simulink model "position_interface"  (R2019b)
settings: Solver=VariableStepAuto  StartTime=0.0  StopTime=10.0  RelTol=1e-3
undefined symbols (not defined in the file or in its folder): Kd, Ki, Kp
settings Model: Creator=AL30832  LastModifiedBy=AL30832

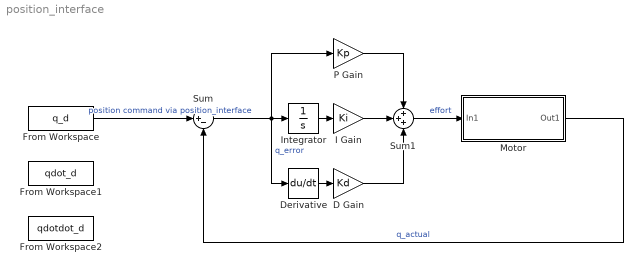
== system position_interface ==
  D Gain : Gain  Gain=Kd
  Derivative : Derivative  CoefficientInTFapproximation=Derivative
  From Workspace : FromWorkspace  VariableName=q_d  SampleTime=0
  From Workspace1 : FromWorkspace  VariableName=qdot_d  SampleTime=0
  From Workspace2 : FromWorkspace  VariableName=qdotdot_d  SampleTime=0
  I Gain : Gain  Gain=Ki
  Integrator : Integrator
  Motor : Subsystem
  P Gain : Gain  Gain=Kp
  Sum : Sum  Inputs=|+-
  Sum1 : Sum  Inputs=+++
  wires:
  From Workspace/1 -> Sum/1  "position command via position_interface"
  Motor/1(Out1) -> Sum/2  "q_actual"
  Sum/1 -> Derivative/1, Integrator/1, P Gain/1  "q_error"
  P Gain/1 -> Sum1/1
  I Gain/1 -> Sum1/2
  D Gain/1 -> Sum1/3
  Sum1/1 -> Motor/1(In1)  "effort"
  Integrator/1 -> I Gain/1
  Derivative/1 -> D Gain/1

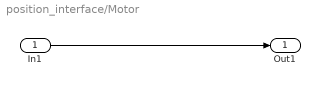
== system position_interface/Motor ==
  In1 : Inport
  Out1 : Outport
  wires:
  In1/1 -> Out1/1
